simulink model "moonOrientation_test"  (R2023b)
settings: Solver=VariableStepAuto  StartTime=0.0  StopTime=time.value  RelTol=1e-3
libraries: dyn_lib x1
settings Model: DataDictionary=Scenario.sldd  Creator=brent  LastModifiedBy=brent

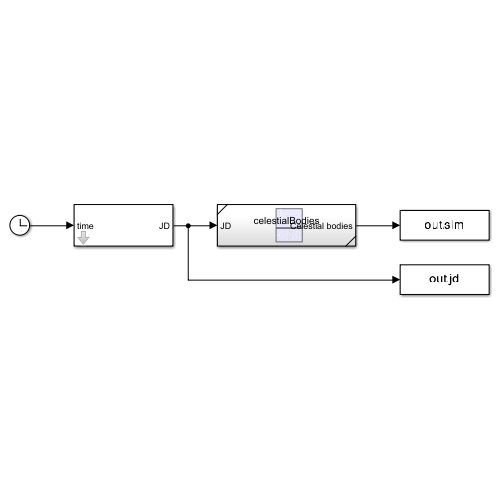
[thumbnail: Simulink's stored preview of the top-level diagram]
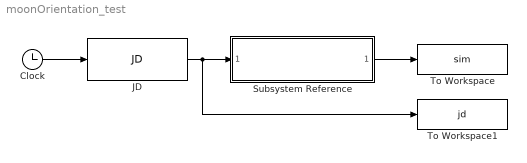
== system moonOrientation_test ==
  Clock : Clock
  JD : dyn_lib/JD  year=Environment.Date.year  month=Environment.Date.month  day=Environment.Date.day  hour=Environment.Date.hour  min=Environment.Date.min  sec=Environment.Date.sec
      settings: SourceProductName=Dynamics library
  Subsystem Reference : Subsystem  ReferencedSubsystem=celestialBodies
      settings: PermitHierarchicalResolution=None
  To Workspace : ToWorkspace  VariableName=sim  SaveFormat=Timeseries  SampleTime=-1
  To Workspace1 : ToWorkspace  VariableName=jd  SaveFormat=Timeseries  SampleTime=-1
  wires:
  JD/1 -> To Workspace1/1, Subsystem Reference/1
  Clock/1 -> JD/1
  Subsystem Reference/1 -> To Workspace/1
